simulink model "VCU_SW_1"  (R2023b)
settings: Solver=FixedStepDiscrete  StartTime=0.0  StopTime=inf  FixedStep=1e-2  RelTol=1e-3
PreLoadFcn:
  | RTWConfigurationCB('preloadfcn', bdroot);
InitFcn:
  | loadvar_ttc500
undefined symbols (not defined in the file): BrkPedalTypes, CabMovModeTypes, cFuseTempSensAcc_X, cFuseTempSensAcc_Y, cFuseTempSensVal_X, cFuseTempSensVal_Y, cTMSTempSensVal_X, cTMSTempSensVal_Y, cTransferCaseSpeedRatio, diag_state, DoorsPositionTypes, dP_filter_Y, DriverOccClassSystemTypes, ErrorValueTypes, fatal_error_callback, IO_ADC_NO_RANGE, LadderStatusTypes, pAnalogCabRotSensAcc, pAnalogCabRotSensMaxVolt, pAnalogCabRotSensMinVolt, pAnalogCabRotSensRange, pAnalogCabRotSensZeroVolt, pBrkActivePress, pCabTiltSensAcc, pCabTiltSensMaxCur, pCabTiltSensMinCur, pDistanceCorrection, pECANManual_BPNEnable, pECANManual_BPNEnabler_Flag, pFilterSensAccRes, pHDirMaxDiffFrq, pHDirSensHighLvl, pHDirSensLowLvl, pMainGearRatio, pMaxFilterSensRes, pMaxFirstPedalSensValue, pMaxFuseTempSensRes, pMaxPressLoss, pMaxPressSensCurrent, pMaxPressValue, pMaxPressValueHydMotAndPump, pMaxPressValueParkDrain, pMaxSecondPedalSensValue, pMaxTempSensVoltage, pMaxTempValue, pMaxTMSTempSensRes, pMinFilterSensRes, pMinFirstPedalSensValue, pMinFuseTempSensRes, pMinPressLoss, pMinPressSensCurrent, pMinPressValue, pMinSecondPedalSensValue, pMinTempSensVoltage, pMinTempValue, pMinTMSTempSensRes, pMotorRingTeethNum, pPedalSensAccuracyPct, pPedalSensAccuracyVolt, pPressLossTreshhold ... (+20)
libraries: TTlibrary x270, canmsglib x127, simulink x88
(part 5 of 19)

== system VCU_SW_1/InputLayer/InputNetwork/InputEngCAN/GetEngCAN100msec ==
  function : TriggerPort  TriggerType=function-call  VariantControl=Variant
  CANUnpack_ECU_EEC1 : canmsglib/CAN Unpack  MsgList=(none)  MsgName=ECU_EEC1  MsgIDType=Extended (29-bit identifier)  MsgIdentifier=217056256  MsgLength=8  SignalInfo={ 'ECU_EEC1_ActEngPTrq', '16', '8', 'LE', 'unsigned', 'Standard', '0', '1', '-125', '-125', '125'; 'ECU_EEC1_ActEngPTrqHighRes', '4', '4', 'LE', 'unsigned', 'Standard', '0', '0.125', '0', '0', '0.875'; 'ECU_EEC1_DrDemEngPTrq', '8', '8', 'LE', 'unsigned', 'Standard', '0', '1', '-125', '-125', '125'; 'ECU_EEC1_EnStrtM', '48', '4', 'LE', 'unsigned', 'Standard', '0', '1', '0', '0', '15'; 'ECU_EEC1_EngDemPercTrq', '56', '8', 'LE', 'unsigned', 'Standard', '0', '1', '-125', '-125', '125'; 'ECU_EEC1_EngSpd', '24', '16', 'LE', 'unsigned', 'Standard', '0', '0.125', '0', '0', '8031.875'; 'ECU_EEC1_EngTrqM', '0', '4', 'LE', 'unsigned', 'Standard', '0', '1', '0', '0', '15'; 'ECU_EEC1_SrsAdr', '40', '8', 'LE', 'unsigned', 'Standard', '0', '1', '0', '0', '255' }  IDPort=off  TimestampPort=off  ErrorPort=off  RemotePort=off  LengthPort=off  StatusPort=off  ApplyMinMax=off
  CANUnpack_ECU_LFE1 : canmsglib/CAN Unpack  MsgList=(none)  MsgName=ECU_LFE1  MsgIDType=Extended (29-bit identifier)  MsgIdentifier=419361280  MsgLength=8  SignalInfo={ 'ECU_LFE1_EngAvrFE', '32', '16', 'LE', 'unsigned', 'Standard', '0', '0.0019531', '0', '0', '125.5'; 'ECU_LFE1_EngFuelRate', '0', '16', 'LE', 'unsigned', 'Standard', '0', '0.05', '0', '0', '3212.75'; 'ECU_LFE1_EngInstFE', '16', '16', 'LE', 'unsigned', 'Standard', '0', '0.0019531', '0', '0', '125.5'; 'ECU_LFE1_EngThrVlv1Pos', '48', '8', 'LE', 'unsigned', 'Standard', '0', '0.4', '0', '0', '100'; 'ECU_LFE1_EngThrVlv2Pos', '56', '8', 'LE', 'unsigned', 'Standard', '0', '0.4', '0', '0', '100' }  IDPort=off  TimestampPort=off  ErrorPort=off  RemotePort=off  LengthPort=off  StatusPort=off  ApplyMinMax=off
  CANUnpack_ECU_TPCM : canmsglib/CAN Unpack  Commented=on  MsgList=(none)  MsgName=ECU_TPCM  MsgIDType=Extended (29-bit identifier)  MsgIdentifier=418184960  MsgLength=8  SignalInfo={ 'ECU_TPCM_ContrByte', '0', '8', 'LE', 'unsigned', 'Standard', '0', '1', '0', '0', '255'; 'ECU_TPCM_MaxNumofPak', '32', '8', 'LE', 'unsigned', 'Standard', '0', '1', '0', '2', '255'; 'ECU_TPCM_NextPakNum', '48', '8', 'LE', 'unsigned', 'Standard', '0', '1', '0', '1', '255'; 'ECU_TPCM_NumPakCanSent', '40', '8', 'LE', 'unsigned', 'Standard', '0', '1', '0', '0', '255'; 'ECU_TPCM_SeqNum', '56', '8', 'LE', 'unsigned', 'Standard', '0', '1', '0', '1', '255'; 'ECU_TPCM_TotMesSize', '8', '16', 'LE', 'unsigned', 'Standard', '0', '1', '0', '9', '1785'; 'ECU_TPCM_TotNumofPak', '24', '8', 'LE', 'unsigned', 'Standard', '0', '1', '0', '2', '255' }  IDPort=off  TimestampPort=off  ErrorPort=off  RemotePort=off  LengthPort=off  StatusPort=off  ApplyMinMax=off
  CANUnpack_ECU_TPDT : canmsglib/CAN Unpack  Commented=on  MsgList=(none)  MsgName=ECU_TPDT  MsgIDType=Extended (29-bit identifier)  MsgIdentifier=418119424  MsgLength=8  SignalInfo={ 'ECU_TPDT_EMS_SeqNum', '0', '8', 'LE', 'unsigned', 'Standard', '0', '1', '0', '1', '255'; 'ECU_TPDT_EMS_byte1', '8', '8', 'LE', 'unsigned', 'Standard', '0', '1', '0', '0', '255'; 'ECU_TPDT_EMS_byte2', '16', '8', 'LE', 'unsigned', 'Standard', '0', '1', '0', '0', '255'; 'ECU_TPDT_EMS_byte3', '24', '8', 'LE', 'unsigned', 'Standard', '0', '1', '0', '0', '255'; 'ECU_TPDT_EMS_byte4', '32', '8', 'LE', 'unsigned', 'Standard', '0', '1', '0', '0', '255'; 'ECU_TPDT_EMS_byte5', '40', '8', 'LE', 'unsigned', 'Standard', '0', '1', '0', '0', '7.20575940379279e+16'; 'ECU_TPDT_EMS_byte6', '48', '8', 'LE', 'unsigned', 'Standard', '0', '1', '0', '0', '255'; 'ECU_TPDT_EMS_byte7', '56', '8', 'LE', 'unsigned', 'Standard', '0', '1', '0', '0', '255' }  IDPort=off  TimestampPort=off  ErrorPort=off  RemotePort=off  LengthPort=off  StatusPort=off  ApplyMinMax=off
  Data Store Write4 : DataStoreWrite  DataStoreName=InputNetworkData  DataStoreElements=InputNetworkData.EngCAN.ActEngPTrq#InputNetworkData.EngCAN.ActEngPTrqHighRes#InputNetworkData.EngCAN.DrDemEngPTrq#InputNetworkData.EngCAN.EnStrtM#InputNetworkData.EngCAN.EngDemPercTrq#InputNetworkData.EngCAN.EngSpd#InputNetworkData.EngCAN.EngTrqM#InputNetworkData.EngCAN.SrsAdr  IndexOptions=Index vector (dialog)  Indices=1  OutputSizes=1
  Data Store Write5 : DataStoreWrite  DataStoreName=InputNetworkData  DataStoreElements=InputNetworkData.EngCAN.EngAvrFE#InputNetworkData.EngCAN.EngFuelRate#InputNetworkData.EngCAN.EngInstFE#InputNetworkData.EngCAN.EngThrVlv1Pos#InputNetworkData.EngCAN.EngThrVlv2Pos  IndexOptions=Index vector (dialog)  Indices=1  OutputSizes=1
  Data Store Write6 : DataStoreWrite  Commented=on  DataStoreName=InputNetworkData  DataStoreElements=InputNetworkData.EngCAN.ContrByte#InputNetworkData.EngCAN.MaxNumofPak#InputNetworkData.EngCAN.NextPakNum#InputNetworkData.EngCAN.NumPakCanSent#InputNetworkData.EngCAN.SeqNum#InputNetworkData.EngCAN.TotMesSize#InputNetworkData.EngCAN.TotNumofPak  IndexOptions=Index vector (dialog)  Indices=1  OutputSizes=1
  Data Store Write7 : DataStoreWrite  Commented=on  DataStoreName=InputNetworkData  DataStoreElements=InputNetworkData.EngCAN.EMS_SeqNum#InputNetworkData.EngCAN.EMS_byte1#InputNetworkData.EngCAN.EMS_byte2#InputNetworkData.EngCAN.EMS_byte3#InputNetworkData.EngCAN.EMS_byte4#InputNetworkData.EngCAN.EMS_byte5#InputNetworkData.EngCAN.EMS_byte6#InputNetworkData.EngCAN.EMS_byte7  IndexOptions=Index vector (dialog)  Indices=1  OutputSizes=1
  Data Type Conversion : DataTypeConversion  OutDataTypeStr=int8  SaturateOnIntegerOverflow=off  RndMeth=Floor
  Data Type Conversion1 : DataTypeConversion  OutDataTypeStr=int8  SaturateOnIntegerOverflow=off  RndMeth=Floor
  Data Type Conversion2 : DataTypeConversion  OutDataTypeStr=int8  SaturateOnIntegerOverflow=off  RndMeth=Floor
  Terminator : Terminator
  Terminator1 : Terminator
  Terminator2 : Terminator  Commented=on
  Terminator3 : Terminator  Commented=on
  calcEnStrtM : MATLAB Function  TreatAsAtomicUnit=on
  read_ECU_EEC1 : TTlibrary/CAN/read_message_name  channel=IO_CAN_CHANNEL_2  id_format=IO_CAN_EXT_FRAME  get_msg_info=off  message_names=there is no CAN Unpack blocks  message_info=|  id=217056256  ac_mask=536870911  retranslation=off  io_error=on  sample_time=-1
      | Message Name: ECU_EEC1
      |  Message ID Type: Extended (29-bit identifier)
      |  Message ID: 217056256
      settings: SourceProductName=TT control 500 series
  read_ECU_LFE1 : TTlibrary/CAN/read_message_name  channel=IO_CAN_CHANNEL_2  id_format=IO_CAN_EXT_FRAME  get_msg_info=off  message_names=there is no CAN Unpack blocks  message_info=|  id=419361280  ac_mask=536870911  retranslation=off  io_error=on  sample_time=-1
      | Message Name: ECU_LFE1
      |  Message ID Type: Extended (29-bit identifier)
      |  Message ID: 419361280
      settings: SourceProductName=TT control 500 series
  read_ECU_TPCM : TTlibrary/CAN/read_message_name  Commented=on  channel=IO_CAN_CHANNEL_2  id_format=IO_CAN_EXT_FRAME  get_msg_info=off  message_names=there is no CAN Unpack blocks  message_info=|  id=418184960  ac_mask=536870911  retranslation=off  io_error=on  sample_time=-1
      | Message Name: ECU_TPCM
      |  Message ID Type: Extended (29-bit identifier)
      |  Message ID: 418184960
      settings: SourceProductName=TT control 500 series
  read_ECU_TPDT : TTlibrary/CAN/read_message_name  Commented=on  channel=IO_CAN_CHANNEL_2  id_format=IO_CAN_EXT_FRAME  get_msg_info=off  message_names=there is no CAN Unpack blocks  message_info=|  id=418119424  ac_mask=536870911  retranslation=off  io_error=on  sample_time=-1
      | Message Name: ECU_TPDT
      |  Message ID Type: Extended (29-bit identifier)
      |  Message ID: 418119424
      settings: SourceProductName=TT control 500 series
  wires:
  CANUnpack_ECU_EEC1/6 -> Data Store Write4/6
  CANUnpack_ECU_EEC1/7 -> Data Store Write4/7
  calcEnStrtM/1(operatingMode) -> Data Store Write4/4
  read_ECU_TPDT/2 -> Terminator3/1  "handler_err_418119424"
  read_ECU_TPCM/2 -> Terminator2/1  "handler_err_418184960"
  read_ECU_LFE1/2 -> Terminator1/1  "handler_err_419361280"
  read_ECU_EEC1/2 -> Terminator/1  "handler_err_217056256"
  CANUnpack_ECU_EEC1/5 -> Data Type Conversion2/1
  CANUnpack_ECU_TPCM/1 -> Data Store Write6/1
  CANUnpack_ECU_EEC1/3 -> Data Type Conversion1/1
  CANUnpack_ECU_TPCM/5 -> Data Store Write6/5
  CANUnpack_ECU_TPDT/3 -> Data Store Write7/3
  CANUnpack_ECU_EEC1/2 -> Data Store Write4/2
  CANUnpack_ECU_TPDT/2 -> Data Store Write7/2
  CANUnpack_ECU_LFE1/2 -> Data Store Write5/2
  CANUnpack_ECU_TPDT/1 -> Data Store Write7/1
  CANUnpack_ECU_TPCM/3 -> Data Store Write6/3
  CANUnpack_ECU_EEC1/4 -> calcEnStrtM/1(Value)
  CANUnpack_ECU_TPDT/6 -> Data Store Write7/6
  CANUnpack_ECU_LFE1/4 -> Data Store Write5/4
  CANUnpack_ECU_TPCM/6 -> Data Store Write6/6
  CANUnpack_ECU_TPCM/2 -> Data Store Write6/2
  CANUnpack_ECU_EEC1/8 -> Data Store Write4/8
  CANUnpack_ECU_TPDT/8 -> Data Store Write7/8
  read_ECU_EEC1/1 -> CANUnpack_ECU_EEC1/1  "msg_217056256"
  CANUnpack_ECU_TPDT/4 -> Data Store Write7/4
  CANUnpack_ECU_TPDT/5 -> Data Store Write7/5
  CANUnpack_ECU_TPCM/4 -> Data Store Write6/4
  CANUnpack_ECU_LFE1/3 -> Data Store Write5/3
  read_ECU_TPCM/1 -> CANUnpack_ECU_TPCM/1  "msg_418184960"
  CANUnpack_ECU_TPDT/7 -> Data Store Write7/7
  CANUnpack_ECU_TPCM/7 -> Data Store Write6/7
  read_ECU_LFE1/1 -> CANUnpack_ECU_LFE1/1  "msg_419361280"
  CANUnpack_ECU_LFE1/5 -> Data Store Write5/5
  CANUnpack_ECU_EEC1/1 -> Data Type Conversion/1
  CANUnpack_ECU_LFE1/1 -> Data Store Write5/1
  read_ECU_TPDT/1 -> CANUnpack_ECU_TPDT/1  "msg_418119424"
  Data Type Conversion/1 -> Data Store Write4/1
  Data Type Conversion1/1 -> Data Store Write4/3
  Data Type Conversion2/1 -> Data Store Write4/5

== system VCU_SW_1/InputLayer/InputNetwork/InputEngCAN/GetEngCAN250msec ==
  function : TriggerPort  TriggerType=function-call  VariantControl=Variant
  CANUnpack_ECU_EEC3 : canmsglib/CAN Unpack  MsgList=(none)  MsgName=ECU_EEC3  MsgIDType=Extended (29-bit identifier)  MsgIdentifier=419356416  MsgLength=8  SignalInfo={ 'ECU_EEC3_Aft1ExDP', '58', '2', 'LE', 'unsigned', 'Standard', '0', '1', '0', '0', '3'; 'ECU_EEC3_Aft1ExGasMasFl', '40', '16', 'LE', 'unsigned', 'Standard', '0', '0.2', '0', '0', '12851'; 'ECU_EEC3_Aft1IntDP', '56', '2', 'LE', 'unsigned', 'Standard', '0', '1', '0', '0', '3'; 'ECU_EEC3_Aft2ExDP', '62', '2', 'LE', 'unsigned', 'Standard', '0', '1', '0', '0', '3'; 'ECU_EEC3_Aft2IntDP', '60', '2', 'LE', 'unsigned', 'Standard', '0', '1', '0', '0', '3'; 'ECU_EEC3_EngDesOpSpd', '8', '16', 'LE', 'unsigned', 'Standard', '0', '0.125', '0', '0', '8031.875'; 'ECU_EEC3_EngDesOpSpdAA', '24', '8', 'LE', 'unsigned', 'Standard', '0', '1', '0', '0', '250'; 'ECU_EEC3_EstEngParLos', '32', '8', 'LE', 'unsigned', 'Standard', '0', '1', '-125', '-125', '125'; 'ECU_EEC3_NomFrPT', '0', '8', 'LE', 'unsigned', 'Standard', '0', '1', '-125', '-125', '125' }  IDPort=off  TimestampPort=off  ErrorPort=off  RemotePort=off  LengthPort=off  StatusPort=off  ApplyMinMax=off
  Data Store Write4 : DataStoreWrite  DataStoreName=InputNetworkData  DataStoreElements=InputNetworkData.EngCAN.Aft1ExDP#InputNetworkData.EngCAN.Aft1ExGasMasFl#InputNetworkData.EngCAN.Aft1IntDP#InputNetworkData.EngCAN.Aft2ExDP#InputNetworkData.EngCAN.Aft2IntDP#InputNetworkData.EngCAN.EngDesOpSpd#InputNetworkData.EngCAN.EngDesOpSpdAA#InputNetworkData.EngCAN.EstEngParLos#InputNetworkData.EngCAN.NomFrPT  IndexOptions=Index vector (dialog)  Indices=1  OutputSizes=1
  Terminator : Terminator
  read_ECU_EEC3 : TTlibrary/CAN/read_message_name  channel=IO_CAN_CHANNEL_2  id_format=IO_CAN_EXT_FRAME  get_msg_info=off  message_names=there is no CAN Unpack blocks  message_info=|  id=419356416  ac_mask=536870911  retranslation=off  io_error=on  sample_time=-1
      | Message Name: ECU_EEC3
      |  Message ID Type: Extended (29-bit identifier)
      |  Message ID: 419356416
      settings: SourceProductName=TT control 500 series
  wires:
  read_ECU_EEC3/2 -> Terminator/1  "handler_err_419356416"
  CANUnpack_ECU_EEC3/2 -> Data Store Write4/2
  read_ECU_EEC3/1 -> CANUnpack_ECU_EEC3/1  "msg_419356416"
  CANUnpack_ECU_EEC3/4 -> Data Store Write4/4
  CANUnpack_ECU_EEC3/7 -> Data Store Write4/7
  CANUnpack_ECU_EEC3/1 -> Data Store Write4/1
  CANUnpack_ECU_EEC3/6 -> Data Store Write4/6
  CANUnpack_ECU_EEC3/9 -> Data Store Write4/9
  CANUnpack_ECU_EEC3/8 -> Data Store Write4/8
  CANUnpack_ECU_EEC3/3 -> Data Store Write4/3
  CANUnpack_ECU_EEC3/5 -> Data Store Write4/5

== system VCU_SW_1/InputLayer/InputNetwork/InputEngCAN/GetEngCAN500msec ==
  function : TriggerPort  TriggerType=function-call  VariantControl=Variant
  CANUnpack_ECU_EFL_P1 : canmsglib/CAN Unpack  MsgList=(none)  MsgName=ECU_EFL_P1  MsgIDType=Extended (29-bit identifier)  MsgIdentifier=419360512  MsgLength=8  SignalInfo={ 'EngCoolLevel', '56', '8', 'LE', 'unsigned', 'Standard', '0', '0.4', '0', '0', '100'; 'EngOilPress', '24', '8', 'LE', 'unsigned', 'Standard', '0', '4', '0', '0', '1000' }  IDPort=off  TimestampPort=off  ErrorPort=off  RemotePort=off  LengthPort=off  StatusPort=off  ApplyMinMax=off
  Data Store Write2 : DataStoreWrite  DataStoreName=InputNetworkData  DataStoreElements=InputNetworkData.EngCAN.EngCoolLevel#InputNetworkData.EngCAN.EngOilPress  IndexOptions=Index vector (dialog)  Indices=1  OutputSizes=1
  Terminator5 : Terminator
  read_ECU_EFL_P1 : TTlibrary/CAN/read_message_name  channel=IO_CAN_CHANNEL_2  id_format=IO_CAN_EXT_FRAME  get_msg_info=off  message_names=there is no CAN Unpack blocks  message_info=|  id=419360512  ac_mask=536870911  retranslation=off  io_error=on  sample_time=-1
      | Message Name: ECU_VEP1
      |  Message ID Type: Extended (29-bit identifier)
      |  Message ID: 419362560
      settings: SourceProductName=TT control 500 series
  wires:
  CANUnpack_ECU_EFL_P1/2 -> Data Store Write2/2
  CANUnpack_ECU_EFL_P1/1 -> Data Store Write2/1
  read_ECU_EFL_P1/2 -> Terminator5/1  "handler_err_419360512"
  read_ECU_EFL_P1/1 -> CANUnpack_ECU_EFL_P1/1  "msg_419360512"

== system VCU_SW_1/InputLayer/InputNetwork/InputEngCAN/GetEngCAN50msec ==
  function : TriggerPort  TriggerType=function-call  VariantControl=Variant
  CANUnpack_ECU_EEC2 : canmsglib/CAN Unpack  MsgList=(none)  MsgName=ECU_EEC2  MsgIDType=Extended (29-bit identifier)  MsgIdentifier=217056000  MsgLength=8  SignalInfo={ 'ECU_EEC2_AccPed1LIS', '0', '2', 'LE', 'unsigned', 'Standard', '0', '1', '0', '0', '3'; 'ECU_EEC2_AccPed2LIS', '6', '2', 'LE', 'unsigned', 'Standard', '0', '1', '0', '0', '3'; 'ECU_EEC2_AccPedKS', '2', '2', 'LE', 'unsigned', 'Standard', '0', '1', '0', '0', '3'; 'ECU_EEC2_AccPedPos1', '8', '8', 'LE', 'unsigned', 'Standard', '0', '0.4', '0', '0', '100'; 'ECU_EEC2_AccPedPos2', '32', '8', 'LE', 'unsigned', 'Standard', '0', '0.4', '0', '0', '100'; 'ECU_EEC2_ActMacAvEngTrq', '48', '8', 'LE', 'unsigned', 'Standard', '0', '0.4', '0', '0', '100'; 'ECU_EEC2_DPF', '44', '2', 'LE', 'unsigned', 'Standard', '0', '1', '0', '0', '3'; 'ECU_EEC2_EngPercLoatCS', '16', '8', 'LE', 'unsigned', 'Standard', '0', '1', '0', '0', '250'; 'ECU_EEC2_EstPumpTrq', '56', '8', 'LE', 'unsigned', 'Standard', '0', '1', '-125', '-125', '125'; 'ECU_EEC2_MomEngMaxPwr', '42', '2', 'LE', 'unsigned', 'Standard', '0', '1', '0', '0', '3'; 'ECU_EEC2_RdSpdLS', '4', '2', 'LE', 'unsigned', 'Standard', '0', '1', '0', '0', '3'; 'ECU_EEC2_RemAccPedPos', '24', '8', 'LE', 'unsigned', 'Standard', '0', '0.4', '0', '0', '100'; 'ECU_EEC2_SCR', '46', '2', 'LE', 'unsigned', 'Standard', '0', '1', '0', '0', '3'; 'ECU_EEC2_VehAccRateLimSts', '40', '2', 'LE', 'unsigned', 'Standard', '0', '1', '0', '0', '3' }  IDPort=off  TimestampPort=off  ErrorPort=off  RemotePort=off  LengthPort=off  StatusPort=off  ApplyMinMax=off
  Data Store Write4 : DataStoreWrite  DataStoreName=InputNetworkData  DataStoreElements=InputNetworkData.EngCAN.AccPed1LIS#InputNetworkData.EngCAN.AccPed2LIS#InputNetworkData.EngCAN.AccPedKS#InputNetworkData.EngCAN.AccPedPos1#InputNetworkData.EngCAN.AccPedPos2#InputNetworkData.EngCAN.ActMacAvEngTrq#InputNetworkData.EngCAN.DPF#InputNetworkData.EngCAN.EngPercLoatCS#InputNetworkData.EngCAN.EstPumpTrq#InputNetworkData.EngCAN.MomEngMaxPwr#InputNetworkData.EngCAN.RdSpdLS#InputNetworkData.EngCAN.RemAccPedPos#InputNetworkData.EngCAN.SCR#InputNetworkData.EngCAN.VehAccRateLimSts  IndexOptions=Index vector (dialog)  Indices=1  OutputSizes=1
  Terminator : Terminator
  read_ECU_EEC2 : TTlibrary/CAN/read_message_name  channel=IO_CAN_CHANNEL_2  id_format=IO_CAN_EXT_FRAME  get_msg_info=off  message_names=there is no CAN Unpack blocks  message_info=|  id=217056000  ac_mask=536870911  retranslation=off  io_error=on  sample_time=-1
      | Message Name: ECU_EEC2
      |  Message ID Type: Extended (29-bit identifier)
      |  Message ID: 217056000
      settings: SourceProductName=TT control 500 series
  wires:
  read_ECU_EEC2/2 -> Terminator/1  "handler_err_217056000"
  CANUnpack_ECU_EEC2/12 -> Data Store Write4/12
  CANUnpack_ECU_EEC2/11 -> Data Store Write4/11
  CANUnpack_ECU_EEC2/13 -> Data Store Write4/13
  CANUnpack_ECU_EEC2/10 -> Data Store Write4/10
  CANUnpack_ECU_EEC2/3 -> Data Store Write4/3
  CANUnpack_ECU_EEC2/8 -> Data Store Write4/8
  CANUnpack_ECU_EEC2/9 -> Data Store Write4/9
  CANUnpack_ECU_EEC2/1 -> Data Store Write4/1
  CANUnpack_ECU_EEC2/4 -> Data Store Write4/4
  CANUnpack_ECU_EEC2/6 -> Data Store Write4/6
  CANUnpack_ECU_EEC2/2 -> Data Store Write4/2
  CANUnpack_ECU_EEC2/14 -> Data Store Write4/14
  CANUnpack_ECU_EEC2/7 -> Data Store Write4/7
  CANUnpack_ECU_EEC2/5 -> Data Store Write4/5
  read_ECU_EEC2/1 -> CANUnpack_ECU_EEC2/1  "msg_217056000"

== system VCU_SW_1/InputLayer/InputNetwork/InputHydCAN/GetHydCAN100msec ==
  function : TriggerPort  TriggerType=function-call  VariantControl=Variant
  Cabine1stLeftHydCylValve : Subsystem
  Cabine2ndRightHydCylValve : Subsystem
  CabineTurningValve : Subsystem

== system VCU_SW_1/InputLayer/InputNetwork/InputStrCAN/Function-Call Subsystem ==
  function : TriggerPort  TriggerType=function-call  VariantControl=Variant
  Data Store Read : DataStoreRead  DataStoreName=InputNetworkData  DataStoreElements=InputNetworkData.StrCAN.joystickNeutralPosStt#InputNetworkData.StrCAN.joystickFwdPosStt#InputNetworkData.StrCAN.joystickBckwdPosStt#InputNetworkData.StrCAN.joystickPct  IndexOptions=Index vector (dialog)  Indices=1  OutputSizes=1
  Data Store Write3 : DataStoreWrite  DataStoreName=InputFunctionsData  DataStoreElements=InputFunctionsData.steerJoyPos  IndexOptions=Index vector (dialog)  Indices=1  OutputSizes=1
  Data Store Write4 : DataStoreWrite  DataStoreName=InputFunctionsData  DataStoreElements=InputFunctionsData.steerJoyDir  IndexOptions=Index vector (dialog)  Indices=1  OutputSizes=1
  MATLAB Function1 : MATLAB Function  TreatAsAtomicUnit=on
  wires:
  MATLAB Function1/1(pos) -> Data Store Write3/1
  MATLAB Function1/2(dir) -> Data Store Write4/1
  Data Store Read/1 -> MATLAB Function1/1(neutralPos)
  Data Store Read/2 -> MATLAB Function1/2(fwdPos)
  Data Store Read/3 -> MATLAB Function1/3(bckwdPos)
  Data Store Read/4 -> MATLAB Function1/4(absPos)

== system VCU_SW_1/InputLayer/InputNetwork/InputStrCAN/GetStrCAN100msec ==
  function : TriggerPort  TriggerType=function-call  VariantControl=Variant
  BJM1 : Subsystem

== system VCU_SW_1/InputLayer/InputNetwork/InputxCraneCAN/GetxCraneCAN100msec ==
  function : TriggerPort  TriggerType=function-call  VariantControl=Variant
  CAN_Unpack_xCrane_PUMPS : canmsglib/CAN Unpack  MsgList=(none)  MsgName=PUMPS  MsgIDType=Extended (29-bit identifier)  MsgIdentifier=218041126  MsgLength=8  SignalInfo={ 'buzzer_req', '58', '2', 'LE', 'unsigned', 'Standard', '0', '1', '0', '0', '3'; 'feeding', '40', '2', 'LE', 'unsigned', 'Standard', '0', '1', '0', '0', '3'; 'feeding_direct', '42', '2', 'LE', 'unsigned', 'Standard', '0', '1', '0', '0', '3'; 'feeding_spd', '44', '2', 'LE', 'unsigned', 'Standard', '0', '1', '0', '0', '3'; 'head_tilt_stt', '48', '2', 'LE', 'unsigned', 'Standard', '0', '1', '0', '0', '3'; 'pump_1_request', '0', '16', 'LE', 'unsigned', 'Standard', '0', '0.016', '0', '0', '1048.56'; 'pump_2_request', '16', '16', 'LE', 'unsigned', 'Standard', '0', '0.016', '0', '0', '1048.56'; 'saw_position', '34', '2', 'LE', 'unsigned', 'Standard', '0', '1', '0', '0', '3'; 'sawing_stt', '32', '2', 'LE', 'unsigned', 'Standard', '0', '1', '0', '0', '3'; 'strump_tratment_req', '56', '2', 'LE', 'unsigned', 'Standard', '0', '1', '0', '0', '3'; 'tilt_stt', '50', '2', 'LE', 'unsigned', 'Standard', '0', '1', '0', '0', '3' }  IDPort=off  TimestampPort=off  ErrorPort=off  RemotePort=off  LengthPort=off  StatusPort=off  ApplyMinMax=off
  DataStoreWrite_xCrane_PUMPS : DataStoreWrite  DataStoreName=InputNetworkData  DataStoreElements=InputNetworkData.xCrCAN.buzzerReq#InputNetworkData.xCrCAN.feeding#InputNetworkData.xCrCAN.feedingDirect#InputNetworkData.xCrCAN.feedingSpeed#InputNetworkData.xCrCAN.headTiltStt#InputNetworkData.xCrCAN.pump1Req#InputNetworkData.xCrCAN.pump2Req#InputNetworkData.xCrCAN.sawPos#InputNetworkData.xCrCAN.sawingStt#InputNetworkData.xCrCAN.strumpTratmentReq#InputNetworkData.xCrCAN.tiltStt  IndexOptions=Index vector (dialog)  Indices=1  OutputSizes=1
  Terminator : Terminator
  read_message_xCrane_PUMPS : TTlibrary/CAN/read_message_name  channel=IO_CAN_CHANNEL_5  id_format=IO_CAN_EXT_FRAME  get_msg_info=off  message_names=there is no CAN Unpack blocks  message_info=|  id=218041126  ac_mask=536870911  retranslation=off  io_error=on  sample_time=-1
      | Message Name: PUMPS
      |  Message ID Type: Extended (29-bit identifier)
      |  Message ID: 218041126
      settings: SourceProductName=TT control 500 series
  wires:
  CAN_Unpack_xCrane_PUMPS/11 -> DataStoreWrite_xCrane_PUMPS/11
  CAN_Unpack_xCrane_PUMPS/10 -> DataStoreWrite_xCrane_PUMPS/10
  CAN_Unpack_xCrane_PUMPS/9 -> DataStoreWrite_xCrane_PUMPS/9
  CAN_Unpack_xCrane_PUMPS/8 -> DataStoreWrite_xCrane_PUMPS/8
  CAN_Unpack_xCrane_PUMPS/7 -> DataStoreWrite_xCrane_PUMPS/7
  CAN_Unpack_xCrane_PUMPS/6 -> DataStoreWrite_xCrane_PUMPS/6
  CAN_Unpack_xCrane_PUMPS/5 -> DataStoreWrite_xCrane_PUMPS/5
  CAN_Unpack_xCrane_PUMPS/4 -> DataStoreWrite_xCrane_PUMPS/4
  CAN_Unpack_xCrane_PUMPS/3 -> DataStoreWrite_xCrane_PUMPS/3
  CAN_Unpack_xCrane_PUMPS/2 -> DataStoreWrite_xCrane_PUMPS/2
  CAN_Unpack_xCrane_PUMPS/1 -> DataStoreWrite_xCrane_PUMPS/1
  read_message_xCrane_PUMPS/2 -> Terminator/1  "handler_err_218041126"
  read_message_xCrane_PUMPS/1 -> CAN_Unpack_xCrane_PUMPS/1  "msg_218041126"

== system VCU_SW_1/InputLayer/Manual/GetManual/Cabin angles + cabin control ==
  Data Store Write1 : DataStoreWrite  DataStoreName=ManualOutputInterfaceData  DataStoreElements=ManualOutputInterfaceData.Cab_Pos_Data_Man.Man_CabineLateralAngle#ManualOutputInterfaceData.Cab_Pos_Data_Man.Man_CabineRotationAngle#ManualOutputInterfaceData.Cab_Pos_Data_Man.Man_CabineTraverseAngle#ManualOutputInterfaceData.Cab_Pos_Data_Man.Man_F_CabineLateralAngle#ManualOutputInterfaceData.Cab_Pos_Data_Man.Man_F_CabineRotationAngle#ManualOutputInterfaceData.Cab_Pos_Data_Man.Man_F_CabineTraverseAngle#ManualOutputInterfaceData.Cab_Pos_Data_Man.Man_F_FrameLateralAngle#ManualOutputInterfaceData.Cab_Pos_Data_Man.Man_F_FrameTraverselAngle#ManualOutputInterfaceData.Cab_Pos_Data_Man.Man_FrameLateralAngle#ManualOutputInterfaceData.Cab_Pos_Data_Man.Man_FrameTraverselAngle#ManualOutputInterfaceData.Cab_Pos_Data_Man.Man_BackwardCabLean_Sts#ManualOutputInterfaceData.Cab_Pos_Data_Man.Man_CabRestoreDefaultRot_Sts#ManualOutputInterfaceData.Cab_Pos_Data_Man.Man_CabRestoreDefaultTilt_Sts#ManualOutputInterfaceData.Cab_Pos_Data_Man.Man_CabStabilization_Sts#ManualOutputInterfaceData.Cab_Pos_Data_Man.Man_F_BackwardCabLean_Sts#ManualOutputInterfaceData.Cab_Pos_Data_Man.Man_F_CabRestoreDefaultRot_Sts#ManualOutputInterfaceData.Cab_Pos_Data_Man.Man_F_CabRestoreDefaultTilt_Sts#ManualOutputInterfaceData.Cab_Pos_Data_Man.Man_F_CabStabilization_Sts#ManualOutputInterfaceData.Cab_Pos_Data_Man.Man_F_ForwardCabLean_Sts#ManualOutputInterfaceData.Cab_Pos_Data_Man.Man_F_LeftCabLean_Sts#ManualOutputInterfaceData.Cab_Pos_Data_Man.Man_F_RightCabLean_Sts#ManualOutputInterfaceData.Cab_Pos_Data_Man.Man_ForwardCabLean_Sts#ManualOutputInterfaceData.Cab_Pos_Data_Man.Man_LeftCabLean_Sts#ManualOutputInterfaceData.Cab_Pos_Data_Man.Man_RightCabLean_Sts  IndexOptions=Index vector (dialog)  Indices=1  OutputSizes=1
  Man_CabineAngles : canmsglib/CAN Unpack  MsgList=(none)  MsgName=Man_CabinAngles  MsgIDType=Extended (29-bit identifier)  MsgIdentifier=402660391  MsgLength=8  SignalInfo={ 'Man_CabineLateralAngle', '0', '8', 'LE', 'unsigned', 'Standard', '0', '0.4', '-50', '-50', '50'; 'Man_CabineRotationAngle', '16', '8', 'LE', 'unsigned', 'Standard', '0', '0.5', '-120', '-120', '120'; 'Man_CabineTraverseAngle', '8', '8', 'LE', 'unsigned', 'Standard', '0', '0.4', '-50', '-50', '50'; 'Man_F_CabineLateralAngle', '40', '1', 'LE', 'unsigned', 'Standard', '0', '1', '0', '0', '1'; 'Man_F_CabineRotationAngle', '42', '1', 'LE', 'unsigned', 'Standard', '0', '1', '0', '0', '1'; 'Man_F_CabineTraverseAngle', '41', '1', 'LE', 'unsigned', 'Standard', '0', '1', '0', '0', '1'; 'Man_F_FrameLateralAngle', '43', '1', 'LE', 'unsigned', 'Standard', '0', '1', '0', '0', '1'; 'Man_F_FrameTraverselAngle', '44', '1', 'LE', 'unsigned', 'Standard', '0', '1', '0', '0', '1'; 'Man_FrameLateralAngle', '24', '8', 'LE', 'unsigned', 'Standard', '0', '0.4', '-50', '-50', '50'; 'Man_FrameTraverselAngle', '32', '8', 'LE', 'unsigned', 'Standard', '0', '0.4', '-50', '-50', '50' }  IDPort=off  TimestampPort=off  ErrorPort=off  RemotePort=off  LengthPort=off  StatusPort=off  ApplyMinMax=off
  Man_CabineControlCommand : canmsglib/CAN Unpack  MsgList=(none)  MsgName=Man_CabineControlCommand  MsgIDType=Extended (29-bit identifier)  MsgIdentifier=402660647  MsgLength=8  SignalInfo={ 'Man_BackwardCabLean_Sts', '0', '2', 'LE', 'unsigned', 'Standard', '0', '1', '0', '0', '3'; 'Man_CabRestoreDefaultRot_Sts', '8', '2', 'LE', 'unsigned', 'Standard', '0', '1', '0', '0', '3'; 'Man_CabRestoreDefaultTilt_Sts', '10', '2', 'LE', 'unsigned', 'Standard', '0', '1', '0', '0', '3'; 'Man_CabStabilization_Sts', '12', '2', 'LE', 'unsigned', 'Standard', '0', '1', '0', '0', '3'; 'Man_F_BackwardCabLean_Sts', '14', '1', 'LE', 'unsigned', 'Standard', '0', '1', '0', '0', '1'; 'Man_F_CabRestoreDefaultRot_Sts', '18', '1', 'LE', 'unsigned', 'Standard', '0', '1', '0', '0', '1'; 'Man_F_CabRestoreDefaultTilt_Sts', '19', '1', 'LE', 'unsigned', 'Standard', '0', '1', '0', '0', '1'; 'Man_F_CabStabilization_Sts', '20', '1', 'LE', 'unsigned', 'Standard', '0', '1', '0', '0', '1'; 'Man_F_ForwardCabLean_Sts', '15', '1', 'LE', 'unsigned', 'Standard', '0', '1', '0', '0', '1'; 'Man_F_LeftCabLean_Sts', '16', '1', 'LE', 'unsigned', 'Standard', '0', '1', '0', '0', '1'; 'Man_F_RightCabLean_Sts', '17', '1', 'LE', 'unsigned', 'Standard', '0', '1', '0', '0', '1'; 'Man_ForwardCabLean_Sts', '2', '2', 'LE', 'unsigned', 'Standard', '0', '1', '0', '0', '3'; 'Man_LeftCabLean_Sts', '4', '2', 'LE', 'unsigned', 'Standard', '0', '1', '0', '0', '3'; 'Man_RightCabLean_Sts', '6', '2', 'LE', 'unsigned', 'Standard', '0', '1', '0', '0', '3' }  IDPort=off  TimestampPort=off  ErrorPort=off  RemotePort=off  LengthPort=off  StatusPort=off  ApplyMinMax=off
  Terminator1 : Terminator
  Terminator2 : Terminator
  read_message_Man_CabineAngles : TTlibrary/CAN/read_message_name  channel=IO_CAN_CHANNEL_6  id_format=IO_CAN_EXT_FRAME  get_msg_info=off  message_names=there is no CAN Unpack blocks  message_info=|  id=4026600391  ac_mask=536870911  retranslation=off  io_error=on  sample_time=-1
      | Message Name: Man_TSC1
      |  Message ID Type: Extended (29-bit identifier)
      |  Message ID: 402659111
      settings: SourceProductName=TT control 500 series
  read_message_Man_CabineControlCommand : TTlibrary/CAN/read_message_name  channel=IO_CAN_CHANNEL_6  id_format=IO_CAN_EXT_FRAME  get_msg_info=off  message_names=there is no CAN Unpack blocks  message_info=|  id=402660647  ac_mask=536870911  retranslation=off  io_error=on  sample_time=-1
      | Message Name: Man_TSC1
      |  Message ID Type: Extended (29-bit identifier)
      |  Message ID: 402659111
      settings: SourceProductName=TT control 500 series
  wires:
  Man_CabineControlCommand/11 -> Data Store Write1/21
  Man_CabineControlCommand/14 -> Data Store Write1/24
  Man_CabineControlCommand/13 -> Data Store Write1/23
  Man_CabineControlCommand/8 -> Data Store Write1/18
  Man_CabineControlCommand/6 -> Data Store Write1/16
  read_message_Man_CabineAngles/2 -> Terminator1/1  "handler_err_4026600391"
  Man_CabineControlCommand/12 -> Data Store Write1/22
  read_message_Man_CabineAngles/1 -> Man_CabineAngles/1  "msg_4026600391"
  Man_CabineAngles/10 -> Data Store Write1/10
  Man_CabineAngles/7 -> Data Store Write1/7
  Man_CabineAngles/5 -> Data Store Write1/5
  Man_CabineControlCommand/5 -> Data Store Write1/15
  Man_CabineAngles/4 -> Data Store Write1/4
  Man_CabineControlCommand/9 -> Data Store Write1/19
  Man_CabineAngles/3 -> Data Store Write1/3
  Man_CabineAngles/2 -> Data Store Write1/2
  Man_CabineControlCommand/10 -> Data Store Write1/20
  Man_CabineAngles/9 -> Data Store Write1/9
  read_message_Man_CabineControlCommand/1 -> Man_CabineControlCommand/1  "msg_402660647"
  Man_CabineControlCommand/3 -> Data Store Write1/13
  Man_CabineAngles/1 -> Data Store Write1/1
  Man_CabineControlCommand/4 -> Data Store Write1/14
  Man_CabineControlCommand/2 -> Data Store Write1/12
  Man_CabineAngles/6 -> Data Store Write1/6
  Man_CabineControlCommand/7 -> Data Store Write1/17
  Man_CabineControlCommand/1 -> Data Store Write1/11
  Man_CabineAngles/8 -> Data Store Write1/8
  read_message_Man_CabineControlCommand/2 -> Terminator2/1  "handler_err_402660647"

== system VCU_SW_1/InputLayer/Manual/GetManual/DO ==
  CAN_ManualData_DO : canmsglib/CAN Unpack  CANdbFile=C:\Work\kora\feature_lightversion\kora\database\ManualParamsCAN.dbc  MsgList=(none)  MsgName=Man_DO  MsgIDType=Extended (29-bit identifier)  MsgIdentifier=402657319  MsgLength=8  SignalInfo={'BrkFrontCircLSVlvSply','16','2','LE','unsigned','Standard','0','1','0','0','3';'BrkLowFluidSensSply','42','2','LE','unsigned','Standard','0','1','0','0','3';'BrkParkCircLSVlvSply','18','2','LE','unsigned','Standard','0','1','0','0','3';'BrkParkCircWorkVlvSply','20','2','LE','unsigned','Standard','0','1','0','0','3';'BrkPressSensSply','24','2','LE','unsigned','Standard','0','1','0','0','3';'BrkRearCircLSVlvSply','22','2','LE','unsigned','Standard','0','1','0','0','3';'BrkSupplyCircPressSensSupply','26','2','LE','unsigned','Standard','0','1','0','0','3';'CabAndPlatformTiltSensSply','58','2','LE','unsigned','Standard','0','1','0','0','3';'CabRotBlockVlvSply','56','2','LE','unsigned','Standard','0','1','0','0','3';'EngAirFilterClogSensSply','38','2','LE','unsigned','Standard','0','1','0','0','3';'EngLowerGenT15','30','2','LE','unsigned','Standard','0','1','0','0','3';'EngPreheaterActivationSig','52','2','LE','unsigned','Standard','0','1','0','0','3';'EngSolenoidRelaySply','34','2','LE','unsigned','Standard','0','1','0','0','3';'EngT15','60','2','LE','unsigned','Standard','0','1','0','0','3';'EngUpperGenT15','28','2','LE','unsigned','Standard','0','1','0','0','3';'ExtrLeftCabPosSensSply','50','2','LE','unsigned','Standard','0','1','0','0','3';'ExtrRightCabCabPosSensSply','54','2','LE','unsigned','Standard','0','1','0','0','3';'FrontAxleDifBlockVlvSply','36','2','LE','unsigned','Standard','0','1','0','0','3';'HydCANDistrSply','14','2','LE','unsigned','Standard','0','1','0','0','3';'IgnitionSwitchPowerSply','48','2','LE','unsigned','Standard','0','1','0','0','3';'RearAxleDifBlockVlvSply','2','2','LE','unsigned','Standard','0','1','0','0','3';'SplyT15','44','2','LE','unsigned','Standard','0','1','0','0','3';'StopLightSensSply','46','2','LE','unsigned','Standard','0','1','0','0','3';'StrAndBrkSysHydPumpDistrSensSply','12','2','LE','unsigned','Standard','0','1','0','0','3';'StrHydDistrSply','32','2','LE','unsigned','Standard','0','1','0','0','3';'TCFrontDrShutoffHydVlvSply','8','2','LE','unsigned','Standard','0','1','0','0','3';'TCGearShiftSensSply','10','2','LE','unsigned','Standard','0','1','0','0','3';'TCHydDistrHighGearVlvSply','6','2','LE','unsigned','Standard','0','1','0','0','3';'TCHydDistrLowGearVlvSply','4','2','LE','unsigned','Standard','0','1','0','0','3';'TechEquipPumpPressSensSply','40','2','LE','unsigned','Standard','0','1','0','0','3';'TrPumpPressLineSensSply','0','2','LE','unsigned','Standard','0','1','0','0','3'}  IDPort=off  TimestampPort=off  ErrorPort=off  RemotePort=off  LengthPort=off  StatusPort=off  ApplyMinMax=off
      settings: DataFormat=CANdb specified signals
  Data Store Write : DataStoreWrite  DataStoreName=ManualOutputInterfaceData  DataStoreElements=ManualOutputInterfaceData.DO_Man.man_frontBrkDistrLSSupply#ManualOutputInterfaceData.DO_Man.man_lowBrakeFluidSensSupply#ManualOutputInterfaceData.DO_Man.man_parkBrkDistrLSSupply#ManualOutputInterfaceData.DO_Man.man_parkBrkDistrSupply#ManualOutputInterfaceData.DO_Man.man_brkSensSupply#ManualOutputInterfaceData.DO_Man.man_rearBrkDistrLSSupply#ManualOutputInterfaceData.DO_Man.man_brkSupplyCircPressSensSupply#ManualOutputInterfaceData.DO_Man.man_cabAndPlatformTiltSensSupply#ManualOutputInterfaceData.DO_Man.man_cabRotBlockVlvSupply#ManualOutputInterfaceData.DO_Man.man_engAirFilterClogSensSupply#ManualOutputInterfaceData.DO_Man.man_lowerGenT15#ManualOutputInterfaceData.DO_Man.man_engPreheaterActivationSig#ManualOutputInterfaceData.DO_Man.man_starterSolenoidCtrl#ManualOutputInterfaceData.DO_Man.man_engT15#ManualOutputInterfaceData.DO_Man.man_upperGenT15#ManualOutputInterfaceData.DO_Man.man_extrLeftCabPosSensSupply#ManualOutputInterfaceData.DO_Man.man_extrRightCabPosSensSupply#ManualOutputInterfaceData.DO_Man.man_frontAxleDifSupply#ManualOutputInterfaceData.DO_Man.man_HydCANPowerSupply#ManualOutputInterfaceData.DO_Man.man_IgnitionSwitchPowerSupply#ManualOutputInterfaceData.DO_Man.man_rearAxleDifSupply#ManualOutputInterfaceData.DO_Man.man_T15_Supply#ManualOutputInterfaceData.DO_Man.man_stopLightSensSupply#ManualOutputInterfaceData.DO_Man.man_strAndBrkPumpDistrSensSupply#ManualOutputInterfaceData.DO_Man.man_steeringDistrSupply#ManualOutputInterfaceData.DO_Man.man_disablingFrontDrDistrSupply#ManualOutputInterfaceData.DO_Man.man_transCaseSensSupply#ManualOutputInterfaceData.DO_Man.man_upperGearDistrTCSupply#ManualOutputInterfaceData.DO_Man.man_lowerGearDistrTCSupply#ManualOutputInterfaceData.DO_Man.man_techEquipPumpPressSensSupply#ManualOutputInterfaceData.DO_Man.man_transPumpPressLinesPressSensSupply  IndexOptions=Index vector (dialog)  Indices=1  OutputSizes=1
  Terminator : Terminator
  read_message_ManualData_DO : TTlibrary/CAN/read_message_name  channel=IO_CAN_CHANNEL_6  id_format=IO_CAN_EXT_FRAME  get_msg_info=off  message_names=there is no CAN Unpack blocks  message_info=|  id=402657319  ac_mask=536870911  retranslation=off  io_error=on  sample_time=-1
      | Message Name: Man_DO
      |  Message ID Type: Extended (29-bit identifier)
      |  Message ID: 402657319
      settings: SourceProductName=TT control 500 series
  wires:
  CAN_ManualData_DO/6 -> Data Store Write/6
  CAN_ManualData_DO/13 -> Data Store Write/13
  CAN_ManualData_DO/21 -> Data Store Write/21
  CAN_ManualData_DO/11 -> Data Store Write/11
  CAN_ManualData_DO/16 -> Data Store Write/16
  CAN_ManualData_DO/1 -> Data Store Write/1
  CAN_ManualData_DO/20 -> Data Store Write/20
  CAN_ManualData_DO/26 -> Data Store Write/26
  CAN_ManualData_DO/19 -> Data Store Write/19
  CAN_ManualData_DO/2 -> Data Store Write/2
  CAN_ManualData_DO/9 -> Data Store Write/9
  CAN_ManualData_DO/22 -> Data Store Write/22
  CAN_ManualData_DO/7 -> Data Store Write/7
  CAN_ManualData_DO/23 -> Data Store Write/23
  CAN_ManualData_DO/18 -> Data Store Write/18
  CAN_ManualData_DO/24 -> Data Store Write/24
  CAN_ManualData_DO/25 -> Data Store Write/25
  CAN_ManualData_DO/28 -> Data Store Write/28
  CAN_ManualData_DO/8 -> Data Store Write/8
  CAN_ManualData_DO/27 -> Data Store Write/27
  CAN_ManualData_DO/10 -> Data Store Write/10
  CAN_ManualData_DO/4 -> Data Store Write/4
  CAN_ManualData_DO/30 -> Data Store Write/30
  CAN_ManualData_DO/29 -> Data Store Write/29
  CAN_ManualData_DO/5 -> Data Store Write/5
  CAN_ManualData_DO/17 -> Data Store Write/17
  CAN_ManualData_DO/31 -> Data Store Write/31
  read_message_ManualData_DO/1 -> CAN_ManualData_DO/1  "msg_402657319"
  CAN_ManualData_DO/3 -> Data Store Write/3
  read_message_ManualData_DO/2 -> Terminator/1  "handler_err_402657319"
  CAN_ManualData_DO/12 -> Data Store Write/12
  CAN_ManualData_DO/14 -> Data Store Write/14
  CAN_ManualData_DO/15 -> Data Store Write/15

== system VCU_SW_1/InputLayer/Manual/GetManual/EEC2 ==
  Data Store Write2 : DataStoreWrite  DataStoreName=ManualOutputInterfaceData  DataStoreElements=ManualOutputInterfaceData.EEC2.Man_AccPedPos1#ManualOutputInterfaceData.EEC2.Man_AccPedPos2#ManualOutputInterfaceData.EEC2.Man_F_AccPedPos1#ManualOutputInterfaceData.EEC2.Man_F_AccPedPos2  IndexOptions=Index vector (dialog)  Indices=1  OutputSizes=1
  Man_EEC2 : canmsglib/CAN Unpack  MsgList=(none)  MsgName=Man_EEC2  MsgIDType=Extended (29-bit identifier)  MsgIdentifier=402660135  MsgLength=8  SignalInfo={ 'Man_AccPedPos1', '0', '8', 'LE', 'unsigned', 'Standard', '0', '0.4', '0', '0', '100'; 'Man_AccPedPos2', '8', '8', 'LE', 'unsigned', 'Standard', '0', '0.4', '0', '0', '100'; 'Man_F_AccPedPos1', '16', '1', 'LE', 'unsigned', 'Standard', '0', '1', '0', '0', '1'; 'Man_F_AccPedPos2', '17', '1', 'LE', 'unsigned', 'Standard', '0', '1', '0', '0', '1' }  IDPort=off  TimestampPort=off  ErrorPort=off  RemotePort=off  LengthPort=off  StatusPort=off  ApplyMinMax=off
  Terminator1 : Terminator
  read_message_Man_EEC2 : TTlibrary/CAN/read_message_name  channel=IO_CAN_CHANNEL_6  id_format=IO_CAN_EXT_FRAME  get_msg_info=off  message_names=there is no CAN Unpack blocks  message_info=|  id=402660135  ac_mask=536870911  retranslation=off  io_error=on  sample_time=-1
      | Message Name: Man_TSC1
      |  Message ID Type: Extended (29-bit identifier)
      |  Message ID: 402659111
      settings: SourceProductName=TT control 500 series
  wires:
  Man_EEC2/1 -> Data Store Write2/1
  Man_EEC2/3 -> Data Store Write2/3
  read_message_Man_EEC2/1 -> Man_EEC2/1  "msg_402660135"
  read_message_Man_EEC2/2 -> Terminator1/1  "handler_err_402660135"
  Man_EEC2/4 -> Data Store Write2/4
  Man_EEC2/2 -> Data Store Write2/2

== system VCU_SW_1/InputLayer/Manual/GetManual/PWM ==
  CAN_ManualData_PWM : canmsglib/CAN Unpack  MsgList=(none)  MsgName=Man_PWM  MsgIDType=Extended (29-bit identifier)  MsgIdentifier=402657575  MsgLength=8  SignalInfo={ 'F_ListenxCraneReqToEquipPump', '50', '2', 'LE', 'unsigned', 'Standard', '0', '1', '0', '0', '3'; 'F_StrAndBrkSysHydPumpSply', '40', '2', 'LE', 'unsigned', 'Standard', '0', '1', '0', '0', '3'; 'F_TechEquipPumpSupply', '42', '2', 'LE', 'unsigned', 'Standard', '0', '1', '0', '0', '3'; 'F_TrHydDistrBackwardMoving', '46', '2', 'LE', 'unsigned', 'Standard', '0', '1', '0', '0', '3'; 'F_TrHydDistrForwardMoving', '44', '2', 'LE', 'unsigned', 'Standard', '0', '1', '0', '0', '3'; 'F_TrHydMotDistrPWMSupply', '48', '2', 'LE', 'unsigned', 'Standard', '0', '1', '0', '0', '3'; 'StrAndBrkSysHydPumpSply', '0', '8', 'LE', 'unsigned', 'Standard', '0', '1', '0', '0', '255'; 'TechEquipPumpSupply', '8', '8', 'LE', 'unsigned', 'Standard', '0', '1', '0', '0', '255'; 'TrHydDistrBackwardMoving', '24', '8', 'LE', 'unsigned', 'Standard', '0', '1', '0', '0', '255'; 'TrHydDistrForwardMoving', '16', '8', 'LE', 'unsigned', 'Standard', '0', '1', '0', '0', '255'; 'TrHydMotDistrPWMSupply', '32', '8', 'LE', 'unsigned', 'Standard', '0', '1', '0', '0', '255'; 'TransPupmpRamp', '56', '8', 'LE', 'unsigned', 'Standard', '0', '1', '0', '0', '255' }  IDPort=off  TimestampPort=off  ErrorPort=off  RemotePort=off  LengthPort=off  StatusPort=off  ApplyMinMax=off
  Data Store Write1 : DataStoreWrite  DataStoreName=ManualOutputInterfaceData  DataStoreElements=ManualOutputInterfaceData.PWM_Man.man_F_ListenxCraneReqToEquipPump#ManualOutputInterfaceData.PWM_Man.man_F_StrAndBrkSysHydPumpSply#ManualOutputInterfaceData.PWM_Man.man_F_TechEquipPumpSupply#ManualOutputInterfaceData.PWM_Man.man_F_TrHydDistrBackwardMoving#ManualOutputInterfaceData.PWM_Man.man_F_TrHydDistrForwardMoving#ManualOutputInterfaceData.PWM_Man.man_F_TrHydMotDistrPWMSupply#ManualOutputInterfaceData.PWM_Man.man_strAndBrkPumpDistrSupply#ManualOutputInterfaceData.PWM_Man.man_techEquipPumpSupply#ManualOutputInterfaceData.PWM_Man.man_reverseTransPumpVlv#ManualOutputInterfaceData.PWM_Man.man_driveTransPumpVlv#ManualOutputInterfaceData.PWM_Man.man_transPumpVlv#ManualOutputInterfaceData.PWM_Man.man_TransPupmpRamp  IndexOptions=Index vector (dialog)  Indices=1  OutputSizes=1
  Terminator1 : Terminator
  read_message_ManualData_PWM : TTlibrary/CAN/read_message_name  channel=IO_CAN_CHANNEL_6  id_format=IO_CAN_EXT_FRAME  get_msg_info=off  message_names=there is no CAN Unpack blocks  message_info=|  id=402657575  ac_mask=536870911  retranslation=off  io_error=on  sample_time=-1
      | Message Name: Man_PWM
      |  Message ID Type: Extended (29-bit identifier)
      |  Message ID: 402657575
      settings: SourceProductName=TT control 500 series
  wires:
  CAN_ManualData_PWM/12 -> Data Store Write1/12
  CAN_ManualData_PWM/11 -> Data Store Write1/11
  CAN_ManualData_PWM/10 -> Data Store Write1/10
  CAN_ManualData_PWM/9 -> Data Store Write1/9
  CAN_ManualData_PWM/8 -> Data Store Write1/8
  CAN_ManualData_PWM/7 -> Data Store Write1/7
  CAN_ManualData_PWM/6 -> Data Store Write1/6
  CAN_ManualData_PWM/5 -> Data Store Write1/5
  CAN_ManualData_PWM/4 -> Data Store Write1/4
  CAN_ManualData_PWM/3 -> Data Store Write1/3
  CAN_ManualData_PWM/1 -> Data Store Write1/1
  read_message_ManualData_PWM/2 -> Terminator1/1  "handler_err_402657575"
  CAN_ManualData_PWM/2 -> Data Store Write1/2
  read_message_ManualData_PWM/1 -> CAN_ManualData_PWM/1  "msg_402657575"

== system VCU_SW_1/InputLayer/Manual/GetManual/Params ==
  CAN_ManualData_Params1 : canmsglib/CAN Unpack  MsgList=(none)  MsgName=Man_Params  MsgIDType=Extended (29-bit identifier)  MsgIdentifier=402658855  MsgLength=8  SignalInfo={ 'Man_AccPedRampSpd', '24', '8', 'LE', 'unsigned', 'Standard', '0', '0.1', '0', '0', '25.5'; 'Man_AccPedalLimit', '16', '8', 'LE', 'unsigned', 'Standard', '0', '1', '0', '0', '255'; 'Man_AccPedalPressed', '7', '1', 'LE', 'unsigned', 'Standard', '0', '1', '0', '0', '1'; 'Man_BrakePedStt', '3', '2', 'LE', 'unsigned', 'Standard', '0', '1', '0', '0', '3'; 'Man_F_AccPedalManualMode', '11', '1', 'LE', 'unsigned', 'Standard', '0', '1', '0', '0', '1'; 'Man_F_BrakePedStt', '10', '1', 'LE', 'unsigned', 'Standard', '0', '1', '0', '0', '1'; 'Man_F_LeverPos', '9', '1', 'LE', 'unsigned', 'Standard', '0', '1', '0', '0', '1'; 'Man_F_PortFlowCmdManip', '62', '1', 'LE', 'unsigned', 'Standard', '0', '1', '0', '0', '1'; 'Man_F_StrCtrl_RunTurning', '8', '1', 'LE', 'unsigned', 'Standard', '0', '1', '0', '0', '1'; 'Man_FailSafeModeCmdManip', '60', '2', 'LE', 'unsigned', 'Standard', '0', '1', '0', '0', '3'; 'Man_LeverPos', '0', '3', 'LE', 'unsigned', 'Standard', '0', '1', '0', '0', '7'; 'Man_PortFlowCmdManip', '48', '8', 'LE', 'unsigned', 'Standard', '0', '1', '0', '0', '100'; 'Man_StrCtrl_LeftTurnBut', '5', '1', 'LE', 'unsigned', 'Standard', '0', '1', '0', '0', '1'; 'Man_StrCtrl_RightTurnBut', '6', '1', 'LE', 'unsigned', 'Standard', '0', '1', '0', '0', '1'; 'Man_Str_OpenVlvLimit', '40', '8', 'LE', 'unsigned', 'Standard', '0', '1', '0', '0', '255'; 'Man_Str_ValveOpenningSpd', '32', '8', 'LE', 'unsigned', 'Standard', '0', '1', '0', '0', '255'; 'Man_ValveStateManip', '56', '4', 'LE', 'unsigned', 'Standard', '0', '1', '0', '0', '15' }  IDPort=off  TimestampPort=off  ErrorPort=off  RemotePort=off  LengthPort=off  StatusPort=off  ApplyMinMax=off
  Data Store Write1 : DataStoreWrite  DataStoreName=ManualOutputInterfaceData  DataStoreElements=ManualOutputInterfaceData.Param_Man.Man_AccPedRampSpd#ManualOutputInterfaceData.Param_Man.Man_AccPedalLimit#ManualOutputInterfaceData.Param_Man.Man_AccPedalPressed#ManualOutputInterfaceData.Param_Man.Man_BrakePedStt#ManualOutputInterfaceData.Param_Man.Man_F_AccPedalManualMode#ManualOutputInterfaceData.Param_Man.Man_F_BrakePedStt#ManualOutputInterfaceData.Param_Man.Man_F_LeverPos#ManualOutputInterfaceData.Param_Man.Man_F_PortFlowCmdManip#ManualOutputInterfaceData.Param_Man.Man_F_StrCtrl_RunTurning#ManualOutputInterfaceData.Param_Man.Man_FailSafeModeCmdManip#ManualOutputInterfaceData.Param_Man.Man_LeverPos#ManualOutputInterfaceData.Param_Man.Man_PortFlowCmdManip#ManualOutputInterfaceData.Param_Man.Man_StrCtrl_LeftTurnBut#ManualOutputInterfaceData.Param_Man.Man_StrCtrl_RightTurnBut#ManualOutputInterfaceData.Param_Man.Man_Str_OpenVlvLimit#ManualOutputInterfaceData.Param_Man.Man_Str_ValveOpenningSpd#ManualOutputInterfaceData.Param_Man.Man_ValveStateManip  IndexOptions=Index vector (dialog)  Indices=1  OutputSizes=1
  Terminator2 : Terminator
  read_message_ManualData_Params : TTlibrary/CAN/read_message_name  channel=IO_CAN_CHANNEL_6  id_format=IO_CAN_EXT_FRAME  get_msg_info=off  message_names=there is no CAN Unpack blocks  message_info=|  id=402658855  ac_mask=536870911  retranslation=off  io_error=on  sample_time=-1
      | Message Name: Man_Params
      |  Message ID Type: Extended (29-bit identifier)
      |  Message ID: 402658855
      settings: SourceProductName=TT control 500 series
  wires:
  CAN_ManualData_Params1/17 -> Data Store Write1/17
  CAN_ManualData_Params1/16 -> Data Store Write1/16
  CAN_ManualData_Params1/15 -> Data Store Write1/15
  CAN_ManualData_Params1/14 -> Data Store Write1/14
  CAN_ManualData_Params1/13 -> Data Store Write1/13
  CAN_ManualData_Params1/12 -> Data Store Write1/12
  CAN_ManualData_Params1/11 -> Data Store Write1/11
  CAN_ManualData_Params1/10 -> Data Store Write1/10
  CAN_ManualData_Params1/9 -> Data Store Write1/9
  CAN_ManualData_Params1/8 -> Data Store Write1/8
  CAN_ManualData_Params1/7 -> Data Store Write1/7
  CAN_ManualData_Params1/6 -> Data Store Write1/6
  CAN_ManualData_Params1/5 -> Data Store Write1/5
  CAN_ManualData_Params1/4 -> Data Store Write1/4
  CAN_ManualData_Params1/3 -> Data Store Write1/3
  CAN_ManualData_Params1/2 -> Data Store Write1/2
  CAN_ManualData_Params1/1 -> Data Store Write1/1
  read_message_ManualData_Params/1 -> CAN_ManualData_Params1/1  "msg_402658855"
  read_message_ManualData_Params/2 -> Terminator2/1  "handler_err_402658855"
